simulink model "simulink_with_sfunction_level2"  (R2017a)
settings: Solver=VariableStepAuto  StartTime=0.0  StopTime=10.0  RelTol=1e-3
settings Model: Creator=veikas  LastModifiedBy=veikas

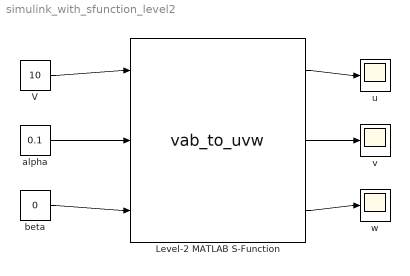
== system simulink_with_sfunction_level2 ==
  Level-2 MATLAB S-Function : M-S-Function  FunctionName=vab_to_uvw
  V : Constant  Value=10
  alpha : Constant  Value=0.1
  beta : Constant  Value=0
  u : Scope
  v : Scope
  w : Scope
  wires:
  V/1 -> Level-2 MATLAB S-Function/1
  alpha/1 -> Level-2 MATLAB S-Function/2
  beta/1 -> Level-2 MATLAB S-Function/3
  Level-2 MATLAB S-Function/3 -> w/1
  Level-2 MATLAB S-Function/2 -> v/1
  Level-2 MATLAB S-Function/1 -> u/1
